simulink model "motor_dc_sim_2022"  (R2022b)
settings: Solver=FixedStepAuto  StartTime=0.0  StopTime=10.0  RelTol=1e-3
values from neighbouring files (symbols this model uses):
  B = 0.1    [motor_dc.m]
  J = 5e-6    (= 5e-06)    [motor_dc.m]
  Ka = 1    [motor_dc.m]
  Kb = 0.5    [motor_dc.m]
  Kc = 1/(2*pi)    (= 0.159154943092)    [motor_dc.m]
  Kt = 1    [motor_dc.m]
  Ra = 50    [motor_dc.m]
settings Model: LastModifiedBy=Fran
settings OptimizationCC: ReuseModelBlockBuffer=on

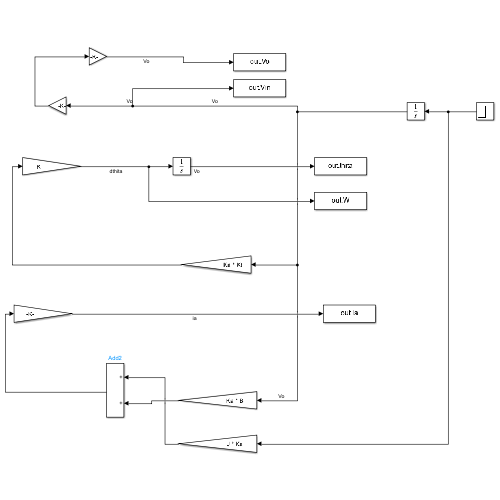
[thumbnail: Simulink's stored preview of the top-level diagram]
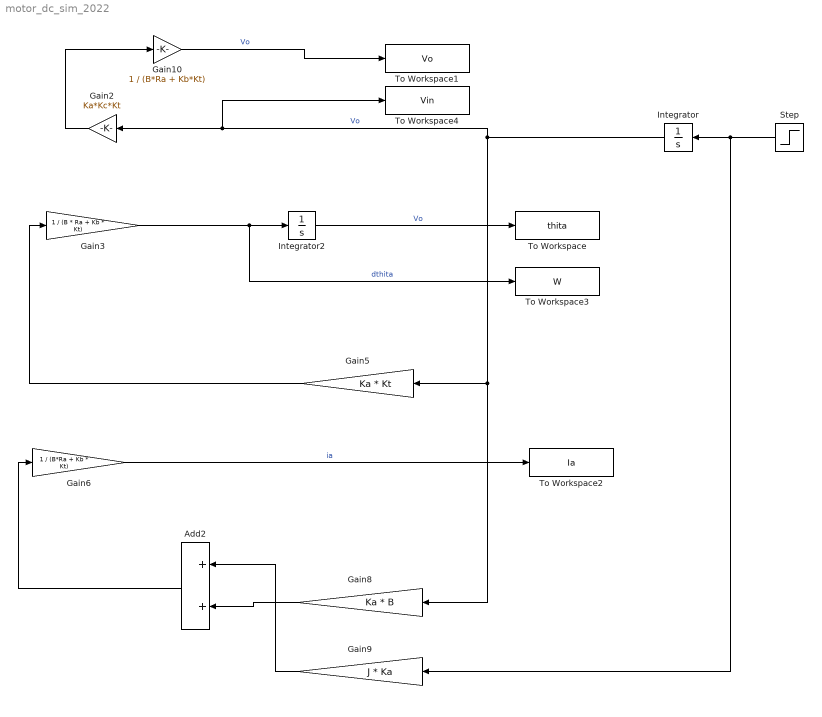
== system motor_dc_sim_2022 ==
  Add2 : Sum
  Gain10 : Gain  Gain=1 / (B*Ra + Kb*Kt)
  Gain2 : Gain  Gain=Ka*Kc*Kt
  Gain3 : Gain  Gain=1 / (B * Ra + Kb * Kt)
  Gain5 : Gain  Gain=Ka * Kt
  Gain6 : Gain  Gain=1 / (B*Ra + Kb * Kt)
  Gain8 : Gain  Gain=Ka * B
  Gain9 : Gain  Gain=J * Ka
  Integrator : Integrator
  Integrator2 : Integrator
  Step : Step  Time=0  SampleTime=0
  To Workspace : ToWorkspace  VariableName=thita  SampleTime=-1
  To Workspace1 : ToWorkspace  VariableName=Vo  SampleTime=-1
  To Workspace2 : ToWorkspace  VariableName=Ia  SampleTime=-1
  To Workspace3 : ToWorkspace  VariableName=W  SampleTime=-1
  To Workspace4 : ToWorkspace  VariableName=Vin  SampleTime=-1
  wires:
  Gain3/1 -> To Workspace3/1, Integrator2/1  "dthita"
  Gain5/1 -> Gain3/1
  Integrator2/1 -> To Workspace/1  "Vo"
  Gain6/1 -> To Workspace2/1  "ia"
  Gain8/1 -> Add2/2
  Add2/1 -> Gain6/1
  Gain9/1 -> Add2/1
  Integrator/1 -> Gain8/1, Gain5/1, Gain2/1, To Workspace4/1  "Vo"
  Gain2/1 -> Gain10/1
  Gain10/1 -> To Workspace1/1  "Vo"
  Step/1 -> Gain9/1, Integrator/1
